simulink model "first"  (R2014a)
settings: Solver=ode15s  StartTime=0.0  StopTime=10.0  MaxStep=1e-3  MinStep=1e-6  RelTol=1e-3
libraries: powerlib x6, simulink x1
settings Model: Creator=EP  LastModifiedBy=EP

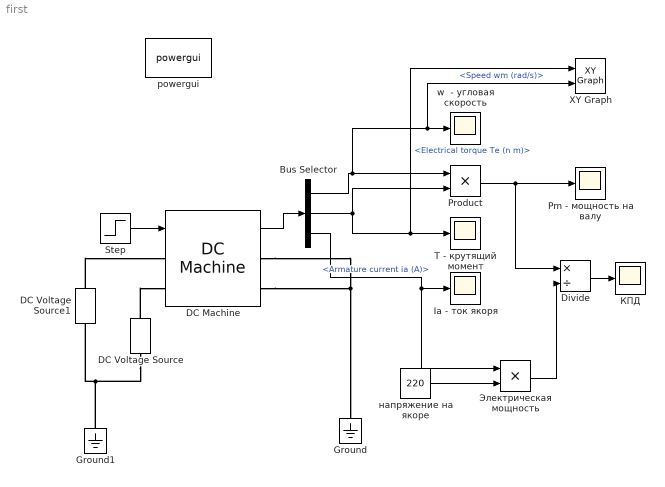
== system first ==
  Bus Selector : BusSelector  OutputSignals=Speed wm (rad/s),Electrical torque Te (n m),Armature current ia (A)
  DC Machine : powerlib/Machines/DC Machine  PresetModel=No  MechanicalLoad=Torque TL  FieldType=Wound  ShowDetailedParameters=on  MeasurementBus=off  RLa=[0.017377 3.52e-4]  RLf=[41.28 9.246e3]  Laf=0.574  MachineConstant=Torque constant (N.m/A)  Ke=1.8  Kt=1.8  J=17  Bm=0  Tf=0  w0=1  Ifinit=1  TsPowergui=0  TsBlock=-1
  DC Voltage Source : powerlib/Electrical Sources/DC Voltage Source  Amplitude=220  Measurements=None
  DC Voltage Source1 : powerlib/Electrical Sources/DC Voltage Source  Amplitude=220  Measurements=None
  Divide : Product  Inputs=*/
  Ground : powerlib/Elements/Ground  LConnTagsString=a
  Ground1 : powerlib/Elements/Ground  LConnTagsString=a
  Ia - ток якоря : Scope
      settings: SaveName=ScopeData2
  Pm - мощность на валу : Scope
      settings: SaveName=ScopeData3
  Product : Product
  Step : Step  After=2171  SampleTime=0
  T - крутящий момент : Scope
  XY Graph : simulink/Sinks/XY Graph  xmin=-5000  xmax=40000  ymin=0  ymax=90  st=-1
  powergui : powerlib/powergui  Priority=1  SimulationMode=Continuous  SolverType=Tustin  SampleTime=50e-6  frequency=60  SPID=off  DisableSnubberDevices=off  DisableRonSwitches=off  DisableVfSwitches=off  SwTol=0  Interpol=off  DisplayEquations=off  Ts=0  methode=off  frequencyindice=0  Pbase=100e6  ErrMax=1e-4  Iterations=50  UnitsV=kV  UnitsW=MW  FunctionMessages=off  echomessages=off  HookPort=off  EnableUseOfTLC=off  x0status=blocks  RestoreLinks=warning  ResistiveCurrentMeasurement=off  Frange=[0:2:500]  Ylog=off  Xlog=on  ShowGrid=off  save=off  variable=ZData  structure=0  ZoomFFT=off  StartTime=0.0  cycles=1  DisplayStyle=1  fundamental=60  FreqAxis=off  MaxFrequency=1000  frequencyindicesteady=1  RmsSteady=1  display=off
  w  - угловая скорость : Scope
  КПД : Scope
      settings: SaveName=ScopeData4
  Электрическая мощность : Product
  напряжение на якоре : Constant  Value=220
  wires:
  DC Machine/1 -> Bus Selector/1
  Bus Selector/1 -> XY Graph/2, w  - угловая скорость/1, Product/1  "<Speed wm (rad/s)>"
  Bus Selector/2 -> Product/2, XY Graph/1, T - крутящий момент/1  "<Electrical torque Te (n m)>"
  Bus Selector/3 -> Электрическая мощность/1, Ia - ток якоря/1  "<Armature current ia (A)>"
  Step/1 -> DC Machine/1
  Product/1 -> Divide/1, Pm - мощность на валу/1
  напряжение на якоре/1 -> Электрическая мощность/2
  Электрическая мощность/1 -> Divide/2
  Divide/1 -> КПД/1
  connections:
  DC Voltage Source/RConn1 -- DC Machine/LConn2
  DC Voltage Source1/RConn1 -- DC Machine/LConn1
  DC Machine/RConn1 -- DC Machine/RConn2 -- Ground/LConn1
  Ground1/LConn1 -- DC Voltage Source1/LConn1 -- DC Voltage Source/LConn1
